simulink library "GPS_time_lib"  (R2016b)
settings: Solver=VariableStepAuto  StartTime=0.0  StopTime=10.0  RelTol=1e-3
undefined symbols (not defined in the file): sim_params
settings Model: Creator=Taylor  LastModifiedBy=Taylor

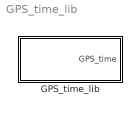
== system GPS_time_lib ==
  GPS_time_lib : Subsystem

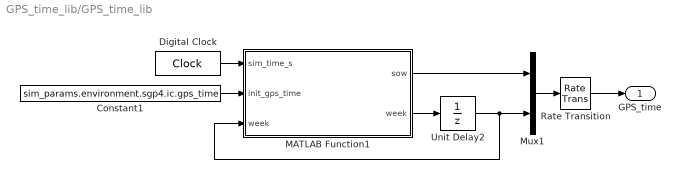
== system GPS_time_lib/GPS_time_lib ==
  Constant1 : Constant  Value=sim_params.environment.sgp4.ic.gps_time  SampleTime=sim_params.sample_time_s
  Digital Clock : DigitalClock  SampleTime=sim_params.sample_time_s
  MATLAB Function1 : MATLAB Function  TreatAsAtomicUnit=on
  Mux1 : Mux  Inputs=2
  Rate Transition : RateTransition  X0=fsw_params.constants.ic.time.gps
  Unit Delay2 : UnitDelay  InitialCondition=sim_params.environment.sgp4.gps_week_init  SampleTime=-1
  GPS_time : Outport
  wires:
  Mux1/1 -> Rate Transition/1
  MATLAB Function1/1(sow) -> Mux1/1
  Unit Delay2/1 -> Mux1/2, MATLAB Function1/3("week ")
  MATLAB Function1/2(week) -> Unit Delay2/1
  Constant1/1 -> MATLAB Function1/2(init_gps_time)
  Digital Clock/1 -> MATLAB Function1/1(sim_time_s)
  Rate Transition/1 -> GPS_time/1

== matlab function GPS_time_lib/MATLAB Function1 ==
  data: sim_time_s input; sow output; init_gps_time input; week input; week output
function [sow, week] = gps_clock(sim_time_s, init_gps_time, week)
% ----------------------------------------------------------------------- %
% UW HuskySat-1, ADCS Subsystem
%
% GPS clock for the SIM.
% ----------------------------------------------------------------------- %

% Constants
sec_in_week = 604800;


init_sow    = init_gps_time(1);
sow         = mod(init_sow + sim_time_s, sec_in_week);

% Handle roll overs
if sow == sec_in_week
    week = week + 1;
end

end
